simulink model "testJacoCommHarness"  (R2017b)
settings: Solver=ode3  StartTime=0.0  StopTime=inf  FixedStep=sampleTime  RelTol=1e-3
PostLoadFcn:
  | q_home = [4.806;2.924;1.004;4.204;1.445;1.323];
  | sampleTime = 0.1;
undefined symbols (not defined in the file or in its folder): JacoCommandModes
libraries: aerolibanimutils x1
settings Model: Creator=csantacr  LastModifiedBy=csantacr
settings SFSimCC: SimUserSources='C:\MATLAB\Demos\robotarm2\Source\Drivers\JACO2Communicator\Source\JacoSDKWrapper.cpp'
settings RTWCC: RTWUseSimCustomCode=on  CustomSource='C:\MATLAB\Demos\robotarm2\Source\Drivers\JACO2Communicator\Source\JacoSDKWrapper.cpp'  Toolchain=Microsoft Visual C++ 2015 v14.0 | nmake (64-bit Windows)  TargetLang=C++
settings CodeAppCC: StateflowObjectComments=on
settings GRTTargetCC: TargetLangStandard=C++03 (ISO)  MultiInstanceERTCode=on  CodeInterfacePackaging=C++ class

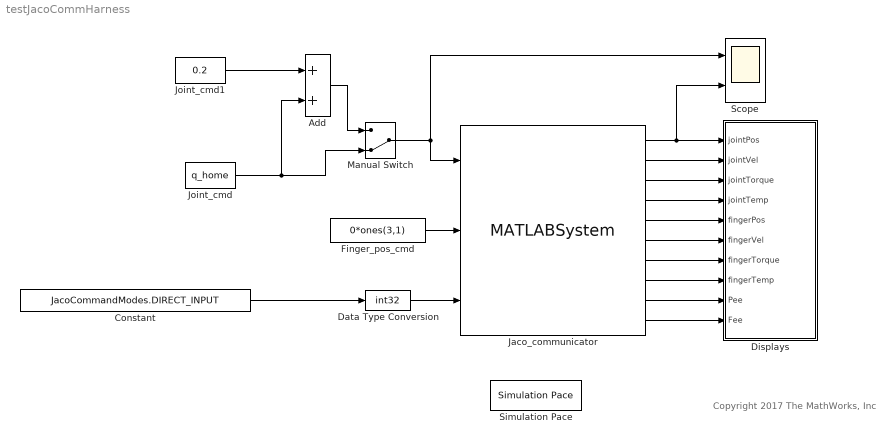
== system testJacoCommHarness ==
  note: Copyright 2017 The MathWorks, Inc
  Add : Sum
  Constant : Constant  Value=JacoCommandModes.DIRECT_INPUT
  Data Type Conversion : DataTypeConversion  OutDataTypeStr=int32
  Displays : Subsystem
  Finger_pos_cmd : Constant  Value=0*ones(3,1)
  Jaco_communicator : MATLABSystem  System=JacoComm  ControlMode=Position  CalibrateFingersAtStartup=off  GoToHomeAtStartup=off  SimulateUsing=Interpreted execution
      mask Type: JacoComm
      mask Display:
      | disp('JacoComm');
      | port_label('input',1,'jnt_pos_cmd');
      | port_label('input',2,'f_cmd');
      | port_label('input',3,'cmd_mode');
      | port_label('output',1,'JointPos');
      | port_label('output',2,'JointVel');
      | port_label('output',3,'JointTorque');
      | port_label('output',4,'JointTemp');
      | port_label('output',5,'FingerPos');
      | port_label('output',6,'FingerVel');
      | port_label('output',7,'FingerTorque');
      | port_label('output',8,'FingerTemp');
      | port_label('output',9,'Pee');
      | port_label('output',10,'Fee');
  Joint_cmd : Constant  Value=q_home  SampleTime=sampleTime
  Joint_cmd1 : Constant  Value=0.2  SampleTime=sampleTime
  Manual Switch : ManualSwitch  CurrentSetting=0
  Scope : Scope  NumInputPorts=2
  Simulation Pace : aerolibanimutils/Simulation Pace  SimulationPace=1  SleepMode=MATLAB Thread  OutputPaceError=off  SampleTime=sampleTime
  wires:
  Jaco_communicator/1 -> Scope/2, Displays/1(jointPos)
  Manual Switch/1 -> Jaco_communicator/1, Scope/1
  Finger_pos_cmd/1 -> Jaco_communicator/2
  Constant/1 -> Data Type Conversion/1
  Joint_cmd/1 -> Add/2, Manual Switch/2
  Add/1 -> Manual Switch/1
  Joint_cmd1/1 -> Add/1
  Jaco_communicator/2 -> Displays/2(jointVel)
  Jaco_communicator/3 -> Displays/3(jointTorque)
  Jaco_communicator/4 -> Displays/4(jointTemp)
  Jaco_communicator/5 -> Displays/5(fingerPos)
  Jaco_communicator/6 -> Displays/6(fingerVel)
  Jaco_communicator/7 -> Displays/7(fingerTorque)
  Jaco_communicator/8 -> Displays/8(fingerTemp)
  Jaco_communicator/9 -> Displays/9(Pee)
  Jaco_communicator/10 -> Displays/10(Fee)
  Data Type Conversion/1 -> Jaco_communicator/3

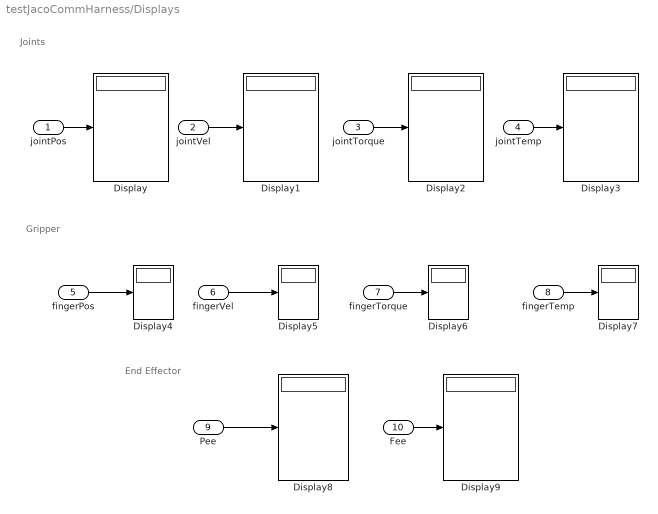
== system testJacoCommHarness/Displays ==
  note: End Effector
  note: Gripper
  note: Joints
  jointPos : Inport
  jointVel : Inport  Port=2
  jointTorque : Inport  Port=3
  jointTemp : Inport  Port=4
  fingerPos : Inport  Port=5
  fingerVel : Inport  Port=6
  fingerTorque : Inport  Port=7
  fingerTemp : Inport  Port=8
  Pee : Inport  Port=9
  Fee : Inport  Port=10
  Display{,1..9} (10 alike) : Display
  wires:
  jointTemp/1 -> Display3/1
  fingerPos/1 -> Display4/1
  fingerVel/1 -> Display5/1
  fingerTorque/1 -> Display6/1
  jointVel/1 -> Display1/1
  jointTorque/1 -> Display2/1
  Fee/1 -> Display9/1
  Pee/1 -> Display8/1
  fingerTemp/1 -> Display7/1
  jointPos/1 -> Display/1
